simulink model "snowpack_water"  (R2014a)
settings: Solver=VariableStepDiscrete  StartTime=0.0  StopTime=10  RelTol=1e-3
model workspace (MAT data in the model file):
  As = 450
  Bs = 20
  Cs = 2.05
  Lf = 334
  Or = 0.01
  Pw = 1000
undefined symbols (not defined in the file): DiscIntNeverNeededParam
settings Model: Creator=feisele  LastModifiedBy=feisele

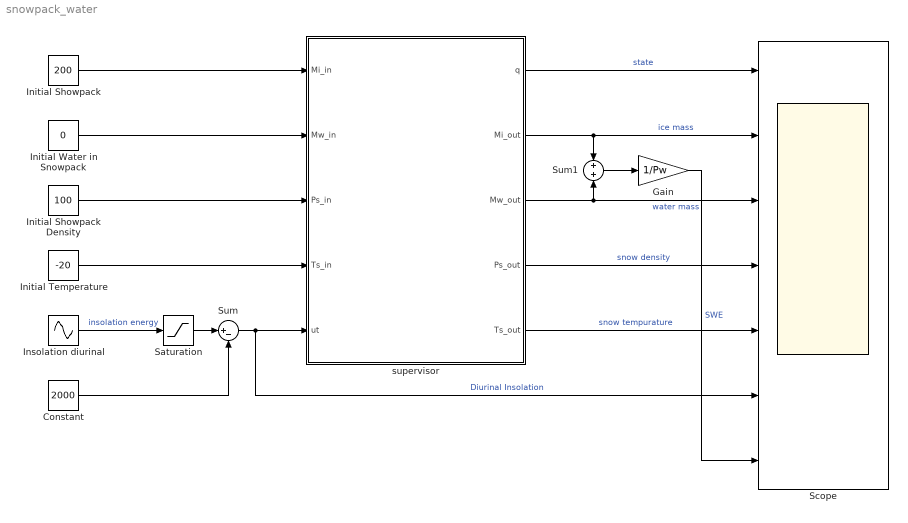
== system snowpack_water ==
  Constant : Constant  Value=2000
  Gain : Gain  Gain=1/Pw
  Initial Showpack : Constant  Value=200
  Initial Showpack Density : Constant  Value=100
  Initial Temperature : Constant  Value=-20
  Initial Water in Snowpack : Constant  Value=0
  Insolation diurinal : Sin  Amplitude=30000  Frequency=2*pi  SampleTime=1/120
  Saturation : Saturate  UpperLimit=inf  LowerLimit=0.0
  Scope : Scope  NumInputPorts=7
      settings: YMin=0~0~0~-1~-25~-20000~0  YMax=4~210~50~200~5~50000~0.3
  Sum : Sum  Inputs=|+-
  Sum1 : Sum  Inputs=+|+
  supervisor : Stateflow chart  TreatAsAtomicUnit=on
  wires:
  Initial Showpack/1 -> supervisor/1(Mi_in)
  Initial Water in Snowpack/1 -> supervisor/2(Mw_in)
  Insolation diurinal/1 -> Saturation/1  "insolation energy"
  Initial Temperature/1 -> supervisor/4(Ts_in)
  Initial Showpack Density/1 -> supervisor/3(Ps_in)
  supervisor/1(q) -> Scope/1  "state"
  supervisor/2(Mi_out) -> Sum1/1, Scope/2  "ice mass"
  supervisor/3(Mw_out) -> Scope/3, Sum1/2  "water mass"
  supervisor/4(Ps_out) -> Scope/4  "snow density"
  supervisor/5(Ts_out) -> Scope/5  "snow tempurature"
  Saturation/1 -> Sum/1
  Sum/1 -> Scope/6, supervisor/5(ut)  "Diurinal Insolation"
  Constant/1 -> Sum/2
  Sum1/1 -> Gain/1
  Gain/1 -> Scope/7  "SWE"

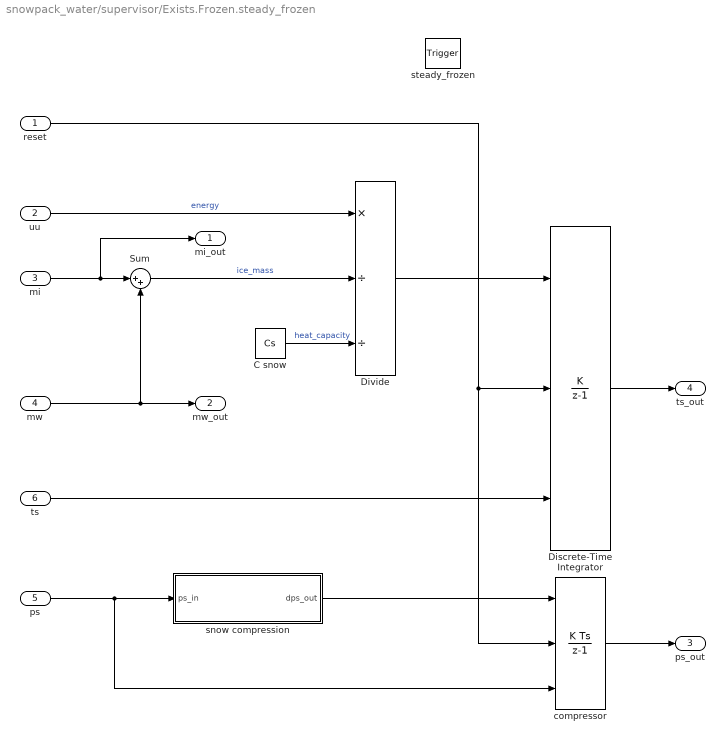
== system snowpack_water/supervisor/Exists.Frozen.steady_frozen ==
  reset : Inport  OutDataTypeStr=double  PortDimensions=1
  uu : Inport  Port=2  OutDataTypeStr=double  PortDimensions=1
  mi : Inport  Port=3  OutDataTypeStr=double  PortDimensions=1
  mw : Inport  Port=4  OutDataTypeStr=double  PortDimensions=1
  ps : Inport  Port=5  OutDataTypeStr=double  PortDimensions=1
  ts : Inport  Port=6  OutDataTypeStr=double  PortDimensions=1
  steady_frozen : TriggerPort  TriggerType=function-call
      settings: CopyFcn=Stateflow.SLINSF.SimulinkMan.removeBlockPreDeleteFcn  PreDeleteFcn=Stateflow.SLINSF.SimulinkMan.unsafePredeleteFcn
  C snow : Constant  Value=Cs
  Discrete-Time Integrator : DiscreteIntegrator  IntegratorMethod=Accumulation: Forward Euler  ExternalReset=rising  InitialConditionSource=external  SampleTime=-1  ICPrevOutput=DiscIntNeverNeededParam  ICPrevScaledInput=DiscIntNeverNeededParam
  Divide : Product  Inputs=*//
  Sum : Sum  Inputs=|++
  compressor : DiscreteIntegrator  ExternalReset=falling  InitialConditionSource=external  SampleTime=-1  ICPrevOutput=DiscIntNeverNeededParam  ICPrevScaledInput=DiscIntNeverNeededParam
  snow compression : MATLAB Function  TreatAsAtomicUnit=on
  mi_out : Outport
  mw_out : Outport  Port=2
  ps_out : Outport  Port=3
  ts_out : Outport  Port=4
  wires:
  Discrete-Time Integrator/1 -> ts_out/1
  Divide/1 -> Discrete-Time Integrator/1
  uu/1 -> Divide/1  "energy"
  ts/1 -> Discrete-Time Integrator/3
  mw/1 -> Sum/2, mw_out/1
  mi/1 -> mi_out/1, Sum/1
  Sum/1 -> Divide/2  "ice_mass"
  ps/1 -> compressor/3, snow compression/1(ps_in)
  C snow/1 -> Divide/3  "heat_capacity"
  snow compression/1(dps_out) -> compressor/1
  compressor/1 -> ps_out/1
  reset/1 -> compressor/2, Discrete-Time Integrator/2

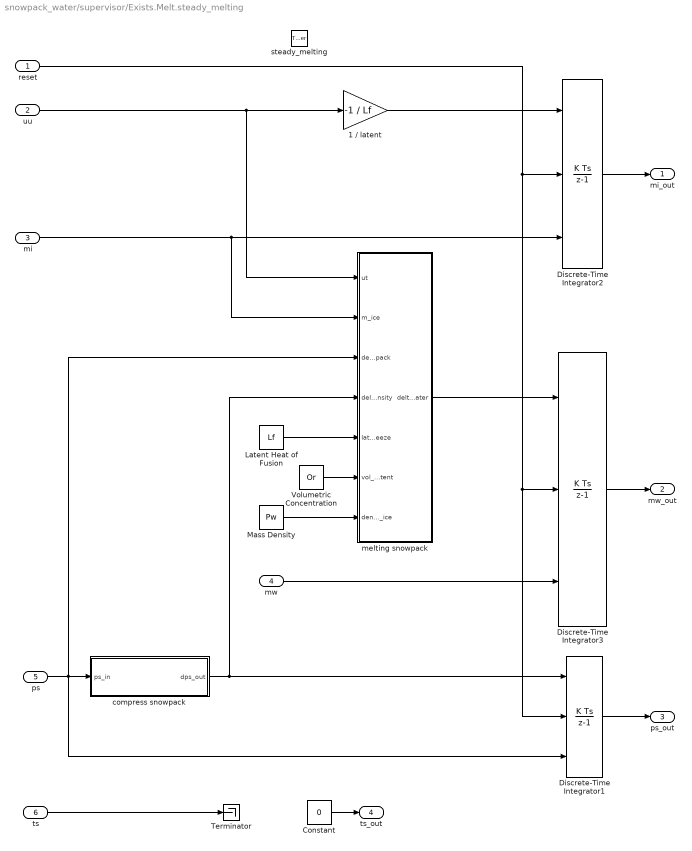
== system snowpack_water/supervisor/Exists.Melt.steady_melting ==
  reset : Inport  OutDataTypeStr=double  PortDimensions=1
  uu : Inport  Port=2  OutDataTypeStr=double  PortDimensions=1
  mi : Inport  Port=3  OutDataTypeStr=double  PortDimensions=1
  mw : Inport  Port=4  OutDataTypeStr=double  PortDimensions=1
  ps : Inport  Port=5  OutDataTypeStr=double  PortDimensions=1
  ts : Inport  Port=6  OutDataTypeStr=double  PortDimensions=1
  steady_melting : TriggerPort  TriggerType=function-call
      settings: CopyFcn=Stateflow.SLINSF.SimulinkMan.removeBlockPreDeleteFcn  PreDeleteFcn=Stateflow.SLINSF.SimulinkMan.unsafePredeleteFcn
  1 / latent : Gain  Gain=-1 / Lf
  Constant : Constant  Value=0
  Discrete-Time Integrator1 : DiscreteIntegrator  ExternalReset=rising  InitialConditionSource=external  SampleTime=-1  ICPrevOutput=DiscIntNeverNeededParam  ICPrevScaledInput=DiscIntNeverNeededParam
  Discrete-Time Integrator2 : DiscreteIntegrator  ExternalReset=rising  InitialConditionSource=external  SampleTime=-1  ICPrevOutput=DiscIntNeverNeededParam  ICPrevScaledInput=DiscIntNeverNeededParam
  Discrete-Time Integrator3 : DiscreteIntegrator  ExternalReset=rising  InitialConditionSource=external  SampleTime=-1  ICPrevOutput=DiscIntNeverNeededParam  ICPrevScaledInput=DiscIntNeverNeededParam
  Latent Heat of Fusion : Constant  Value=Lf
  Mass Density : Constant  Value=Pw
  Terminator : Terminator
  Volumetric Concentration : Constant  Value=Or
  compress snowpack : MATLAB Function  TreatAsAtomicUnit=on
  melting snowpack : MATLAB Function  TreatAsAtomicUnit=on
  mi_out : Outport
  mw_out : Outport  Port=2
  ps_out : Outport  Port=3
  ts_out : Outport  Port=4
  wires:
  uu/1 -> melting snowpack/1(ut), 1 / latent/1
  ts/1 -> Terminator/1
  mi/1 -> Discrete-Time Integrator2/3, melting snowpack/2(m_ice)
  Discrete-Time Integrator2/1 -> mi_out/1
  1 / latent/1 -> Discrete-Time Integrator2/1
  mw/1 -> Discrete-Time Integrator3/3
  Discrete-Time Integrator3/1 -> mw_out/1
  Constant/1 -> ts_out/1
  compress snowpack/1(dps_out) -> Discrete-Time Integrator1/1, melting snowpack/4(delta_density)
  ps/1 -> Discrete-Time Integrator1/3, melting snowpack/3(density_snowpack), compress snowpack/1(ps_in)
  melting snowpack/1(delta_mass_water) -> Discrete-Time Integrator3/1
  Latent Heat of Fusion/1 -> melting snowpack/5(latent_freeze)
  Volumetric Concentration/1 -> melting snowpack/6(vol_content)
  Mass Density/1 -> melting snowpack/7(density_ice)
  Discrete-Time Integrator1/1 -> ps_out/1
  reset/1 -> Discrete-Time Integrator1/2, Discrete-Time Integrator3/2, Discrete-Time Integrator2/2

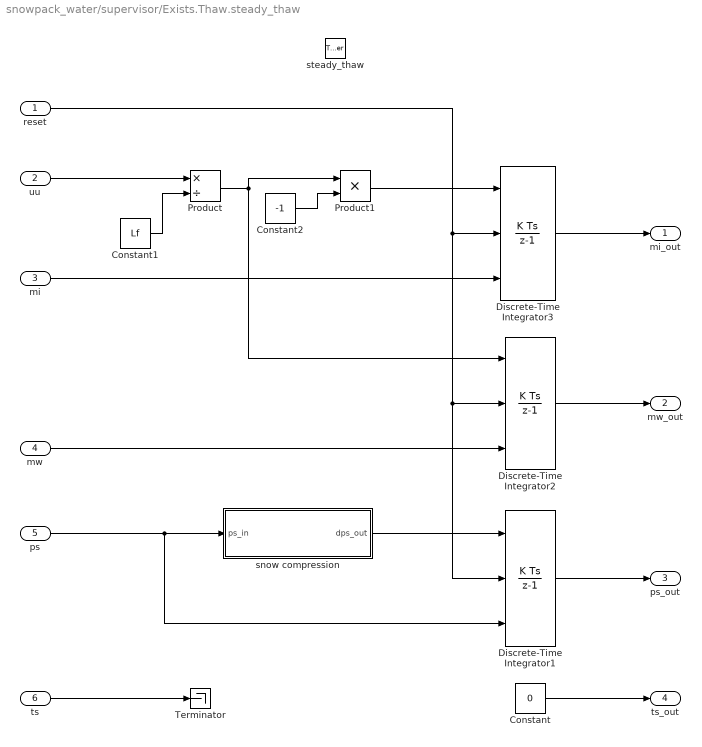
== system snowpack_water/supervisor/Exists.Thaw.steady_thaw ==
  reset : Inport  OutDataTypeStr=double  PortDimensions=1
  uu : Inport  Port=2  OutDataTypeStr=double  PortDimensions=1
  mi : Inport  Port=3  OutDataTypeStr=double  PortDimensions=1
  mw : Inport  Port=4  OutDataTypeStr=double  PortDimensions=1
  ps : Inport  Port=5  OutDataTypeStr=double  PortDimensions=1
  ts : Inport  Port=6  OutDataTypeStr=double  PortDimensions=1
  steady_thaw : TriggerPort  TriggerType=function-call
      settings: CopyFcn=Stateflow.SLINSF.SimulinkMan.removeBlockPreDeleteFcn  PreDeleteFcn=Stateflow.SLINSF.SimulinkMan.unsafePredeleteFcn
  Constant : Constant  Value=0
  Constant1 : Constant  Value=Lf
  Constant2 : Constant  Value=-1
  Discrete-Time Integrator1 : DiscreteIntegrator  ExternalReset=rising  InitialConditionSource=external  SampleTime=-1  ICPrevOutput=DiscIntNeverNeededParam  ICPrevScaledInput=DiscIntNeverNeededParam
  Discrete-Time Integrator2 : DiscreteIntegrator  ExternalReset=rising  InitialConditionSource=external  SampleTime=-1  ICPrevOutput=DiscIntNeverNeededParam  ICPrevScaledInput=DiscIntNeverNeededParam
  Discrete-Time Integrator3 : DiscreteIntegrator  ExternalReset=either  InitialConditionSource=external  SampleTime=-1  ICPrevOutput=DiscIntNeverNeededParam  ICPrevScaledInput=DiscIntNeverNeededParam
  Product : Product  Inputs=*/
  Product1 : Product  Inputs=**
  Terminator : Terminator
  snow compression : MATLAB Function  TreatAsAtomicUnit=on
  mi_out : Outport
  mw_out : Outport  Port=2
  ps_out : Outport  Port=3
  ts_out : Outport  Port=4
  wires:
  mi/1 -> Discrete-Time Integrator3/3
  Discrete-Time Integrator3/1 -> mi_out/1
  mw/1 -> Discrete-Time Integrator2/3
  Discrete-Time Integrator2/1 -> mw_out/1
  ts/1 -> Terminator/1
  Constant/1 -> ts_out/1
  ps/1 -> Discrete-Time Integrator1/3, snow compression/1(ps_in)
  snow compression/1(dps_out) -> Discrete-Time Integrator1/1
  Discrete-Time Integrator1/1 -> ps_out/1
  reset/1 -> Discrete-Time Integrator1/2, Discrete-Time Integrator2/2, Discrete-Time Integrator3/2
  Constant1/1 -> Product/2
  uu/1 -> Product/1
  Product/1 -> Product1/1, Discrete-Time Integrator2/1
  Product1/1 -> Discrete-Time Integrator3/1
  Constant2/1 -> Product1/2

== matlab function snowpack_water/supervisor/Exists.Melt.steady_melting/compress snowpack ==
  data: ps_in input; dps_out output
function dps_out = snow_compression(ps_in)
%#codegen
As = 450;
Bs = 20; % days
ratio = 1 + (ps_in / (As - ps_in));
dps_out = As / (Bs * ratio * ratio);

== matlab function snowpack_water/supervisor/Exists.Frozen.steady_frozen/snow compression ==
  data: ps_in input; dps_out output
function dps_out = snow_compression(ps_in)
%#codegen
As = 450;
Bs = 20; % days
ratio = 1 + (ps_in / (As - ps_in));
dps_out = As / (Bs * ratio * ratio);

== stateflow chart snowpack_water/supervisor ==
  state Exists/
    state Frozen/
      entry:
      [Mi, Mw, Ps, Ts] = steady_frozen(1, ut, Mi, Mw, Ps, Ts);
      during:
      q = 1;
      [Mi, Mw, Ps, Ts] = steady_frozen(0, ut, Mi, Mw, Ps, Ts);
      Mi_out = Mi;
      Mw_out = Mw;
      Ps_out = Ps;
      Ts_out = Ts;
      state [mi_out,mw_out,ps_out,ts_out] = steady_frozen(reset,uu,mi,mw,ps,ts) [function]
    state Thaw/
      entry:
      [Mi, Mw, Ps, Ts] = steady_thaw(1, ut, Mi, Mw, Ps, Ts);
      during:
      q = 2;
      [Mi, Mw, Ps, Ts] = steady_thaw(0, ut, Mi, Mw, Ps, Ts);
      Mi_out = Mi;
      Mw_out = Mw;
      Ps_out = Ps;
      Ts_out = Ts;
      state [mi_out,mw_out,ps_out,ts_out] = steady_thaw(reset,uu,mi,mw,ps,ts) [function]
    state Melt/
      entry:
      [Mi, Mw, Ps, Ts] = steady_melting(1, ut, Mi, Mw, Ps, Ts);
      during:
      q = 3;
      [Mi, Mw, Ps, Ts] = steady_melting(0, ut, Mi, Mw, Ps, Ts);
      Mi_out = Mi;
      Mw_out = Mw;
      Ps_out = Ps;
      Ts_out = Ts;
      state [mi_out,mw_out,ps_out,ts_out] = steady_melting(reset, uu,mi,mw,ps,ts) [function]
    (default) -> Frozen : {
        | q = 0;
        | Mi = Mi_in;
        | Mi_out = Mi_in;
        | Mw = Mw_in;
        | Mw_out = Mw_in;
        | Ps = Ps_in;
        | Ps_out = Ps_in;
        | Ts = Ts_in;
        | Ts_out = Ts_in;
        | }
      settings: description=Generally, when snow falls the T is <= 0 degrees C, the density is some initial value and there is no liquid water present, all ice.
    Thaw -> Frozen [order 2] : [q == 2 && Mw <= 0]
      settings: description=Once all the water has frozen; there is no more liquid water, the frozen state is entered.
    Frozen -> Thaw : [q == 1 && Ts >= 0]
      settings: description=The isothermal region is reached, T = 0 degrees C.
    Melt -> Thaw : [q == 3 && (Ps * Mw) / (Pw * (Mi + Mw)) < Or]
      settings: description=When the water content, Ow, of the snowpack reache a value lower than the adsorbtion threshold, Or, water ceases to melt from the system.
    Thaw -> Melt [order 1] : [q == 2 &&  (Ps * Mw) / (Pw * (Mi + Mw)) >= Or]
      settings: description=When the water content, Ow, of the snowpack reaches a value greater than or equal to the adsorbtion threshold, Or, water begins to leave the system; melting begins.
  state Exhausted/
    entry:
    q = 0;
    Mi_out = 0;
    Mw_out = 0;
    Ps_out = 0;
    Ts_out = 0;
  (default) -> Exists
  Exists -> Exhausted : [Mi <= 0]
  Exhausted -> Exists : [Mi > 0]
  data: reset function_input double size=1; mi_out function_output; mw_out function_output; ps_out function_output; ts_out function_output; uu function_input double size=1; mi function_input double size=1; mw function_input double size=1; ps function_input double size=1; ts function_input double size=1; reset function_input double size=1; uu function_input double size=1; mi function_input double size=1; mw function_input double size=1; ps function_input double size=1; ts function_input double size=1; mi_out function_output; mw_out function_output; ps_out function_output; ts_out function_output; reset function_input double size=1; mi_out function_output; mw_out function_output; ps_out function_output; ts_out function_output; uu function_input double size=1; mi function_input double size=1; mw function_input double size=1; ps function_input double size=1; ts function_input double size=1; q output double; Mi_in input double; Mw_in input double; Ps_in input double; Ts_in input double; Mi_out output double; Mw_out output double; Ps_out output double; Ts_out output double; ut input double; Mi local double; Mw local double; Ps local double; Ts local double; Pw constant double =1000; Or constant double =0.01
  data q settings: description=|
      | An integer indicating the supervisor mode:
      | 1 : Frozen : Sub-freezing temperature, all solid
      | 2 : Thawing : Iso-thermal, a mixure of liquid and water but liquid is absorbed by the solid portion.
      | 3 : Melting : Iso-thermal, a mixture of liquid and solid but with an excess of liquid.
  data Mi_in settings: description=The mass of ice in the snowpack
  data ut settings: description=The amount of energy introduced to the system.
  data Mi settings: updateMethod=SF_CONTINUOUS_TIME_DATA  description=Current mass of ice (solid) in the snowpack.
  data Mw settings: updateMethod=SF_CONTINUOUS_TIME_DATA  description=Current mass of the water (liquid) in the snowpack
  data Ps settings: updateMethod=SF_CONTINUOUS_TIME_DATA  description=Current density of the snow.
  data Ts settings: updateMethod=SF_CONTINUOUS_TIME_DATA  description=Buld tempurature of the snow pack

== matlab function snowpack_water/supervisor/Exists.Thaw.steady_thaw/snow compression ==
  data: ps_in input; dps_out output
function dps_out = snow_compression(ps_in)
%#codegen
As = 450;
Bs = 20; % days
ratio = 1 + (ps_in / (As - ps_in));
dps_out = As / (Bs * ratio * ratio);

== matlab function snowpack_water/supervisor/Exists.Melt.steady_melting/melting snowpack ==
  data: ut input; m_ice input; delta_mass_water output; density_snowpack input; delta_density input; latent_freeze input; vol_content input; density_ice input
function delta_mass_water = snow_melter(ut, m_ice, density_snowpack, delta_density, ...
      latent_freeze, vol_content, density_ice)
%SNOW_MELTER determine the change in water in the snowpack.
reduction = ut / latent_freeze ...
    * ((vol_content * density_ice) - density_snowpack) ...
    - m_ice * delta_density;
vol_density = vol_content * density_ice;
delta_mass_water = (vol_density * reduction) / ...
            (density_snowpack - vol_density)^2;
